simulink model "IFSSIM_Plant"  (R2025b)
settings: Solver=ode1  StartTime=0  StopTime=inf  FixedStep=0.0010416666666666671  RelTol=1e-3
undefined symbols (not defined in the file or in its folder): IFSSIM_PoseBus_init
settings Model: Creator=raulmoran  LastModifiedBy=raulmoran

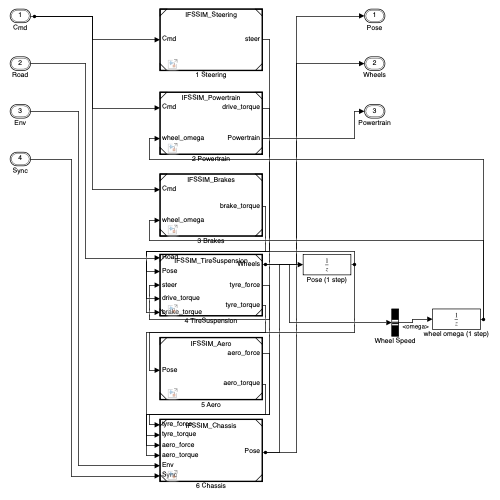
[thumbnail: Simulink's stored preview of the top-level diagram]
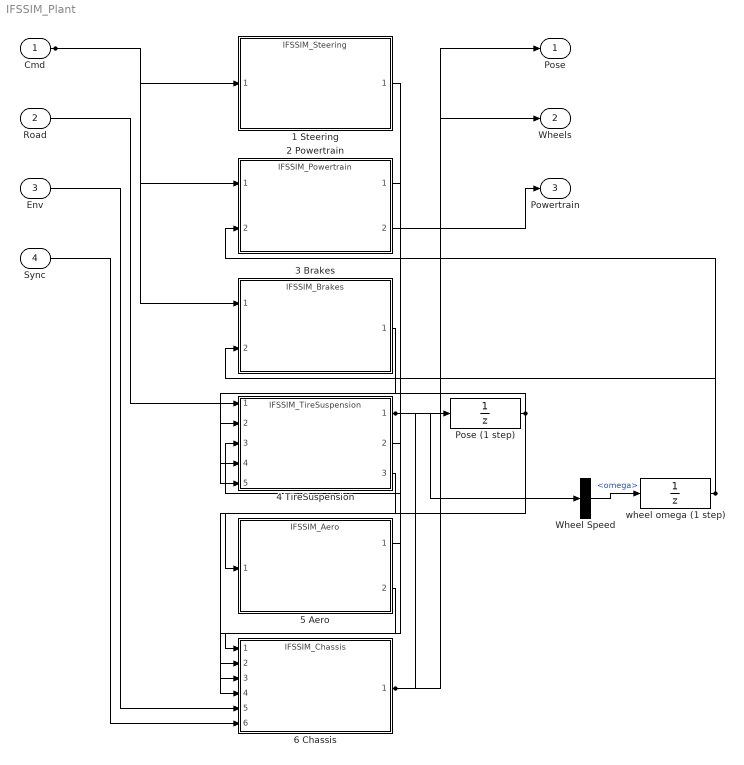
== system IFSSIM_Plant ==
  Cmd : Inport  OutDataTypeStr=Bus: IFSSIM_CmdBus  BusOutputAsStruct=on
  Road : Inport  Port=2  OutDataTypeStr=Bus: IFSSIM_RoadBus  BusOutputAsStruct=on
  Env : Inport  Port=3  OutDataTypeStr=Bus: IFSSIM_EnvBus  BusOutputAsStruct=on
  Sync : Inport  Port=4  OutDataTypeStr=Bus: IFSSIM_SyncBus  BusOutputAsStruct=on
  1 Steering : ModelReference  ModelNameDialog=IFSSIM_Steering.slx  SimulationMode=Normal  ModelReferenceVersion=1.1
  2 Powertrain : ModelReference  ModelNameDialog=IFSSIM_Powertrain.slx  SimulationMode=Normal  ModelReferenceVersion=1.1
  3 Brakes : ModelReference  ModelNameDialog=IFSSIM_Brakes.slx  SimulationMode=Normal  ModelReferenceVersion=1.1
  4 TireSuspension : ModelReference  ModelNameDialog=IFSSIM_TireSuspension.slx  SimulationMode=Normal  ModelReferenceVersion=1.1
  5 Aero : ModelReference  ModelNameDialog=IFSSIM_Aero.slx  SimulationMode=Normal  ModelReferenceVersion=1.1
  6 Chassis : ModelReference  ModelNameDialog=IFSSIM_Chassis.slx  SimulationMode=Normal  ModelReferenceVersion=1.1
  Pose (1 step) : UnitDelay  InitialCondition=IFSSIM_PoseBus_init  SampleTime=-1  HasFrameUpgradeWarning=on
  Wheel Speed : BusSelector  OutputSignals=omega
  wheel omega (1 step) : UnitDelay  InitialCondition=[0;0;0;0]  SampleTime=-1  HasFrameUpgradeWarning=on
  Pose : Outport  OutDataTypeStr=Bus: IFSSIM_PoseBus
  Wheels : Outport  Port=2  OutDataTypeStr=Bus: IFSSIM_WheelsBus
  Powertrain : Outport  Port=3  OutDataTypeStr=Bus: IFSSIM_PowertrainBus
  wires:
  Cmd/1 -> 1 Steering/1, 2 Powertrain/1, 3 Brakes/1
  Road/1 -> 4 TireSuspension/1
  Env/1 -> 6 Chassis/5
  Sync/1 -> 6 Chassis/6
  1 Steering/1 -> 4 TireSuspension/3
  2 Powertrain/1 -> 4 TireSuspension/4
  3 Brakes/1 -> 4 TireSuspension/5
  4 TireSuspension/2 -> 6 Chassis/1
  4 TireSuspension/3 -> 6 Chassis/2
  5 Aero/1 -> 6 Chassis/3
  5 Aero/2 -> 6 Chassis/4
  6 Chassis/1 -> Pose/1, Pose (1 step)/1
  4 TireSuspension/1 -> Wheels/1, Wheel Speed/1
  2 Powertrain/2 -> Powertrain/1
  Pose (1 step)/1 -> 4 TireSuspension/2, 5 Aero/1
  Wheel Speed/1 -> wheel omega (1 step)/1  "<omega>"
  wheel omega (1 step)/1 -> 2 Powertrain/2, 3 Brakes/2
